simulink model "Echangeur_chaleur"  (R2020b)
settings: Solver=VariableStepAuto  StartTime=0.0  StopTime=10.0  RelTol=1e-3
values from neighbouring files (symbols this model uses):
  d_tube_big_ext = 0.106    [Conception_Preliminaire.m]    (also in Main.m)
  d_tube_big_int = 0.08    [Conception_Preliminaire.m]    (also in Main.m)
  d_tube_moy_ext = 0.01    [Conception_Preliminaire.m]    (also in Main.m)
  d_tube_moy_int = 0.007    [Conception_Preliminaire.m]    (also in Main.m)
  d_tube_small_ext = 0.006    [Conception_Preliminaire.m]    (also in Main.m)
  d_tube_small_int = 0.004    [Conception_Preliminaire.m]    (also in Main.m)
  h_int_MDI = 4.452    [Conception_Preliminaire.m]    (also in Main.m)
  k_acier = 36    [Conception_Preliminaire.m]    (also in Dimensionnement.m; Main.m)
  k_H2O = 0.147    [Conception_Preliminaire.m]    (also in Dimensionnement.m; Main.m)
  k_MDI = 0.08648    [Conception_Preliminaire.m]    (also in Dimensionnement.m; Main.m)
  L = 3    [Dimensionnement.m]    (also in Main.m = 2.72)
  Pr_H2O = 70    [Conception_Preliminaire.m]    (also in Main.m)
  Pr_lam_plaque_MDI = 10    [Conception_Preliminaire.m]    (also in Main.m)
  visc_H2O = 0.042    [Conception_Preliminaire.m]    (also in Dimensionnement.m; Main.m)
  visc_MDI = 0.19    [Conception_Preliminaire.m]    (also in Dimensionnement.m; Main.m)
settings Model: Creator=sam_f  LastModifiedBy=sam_f

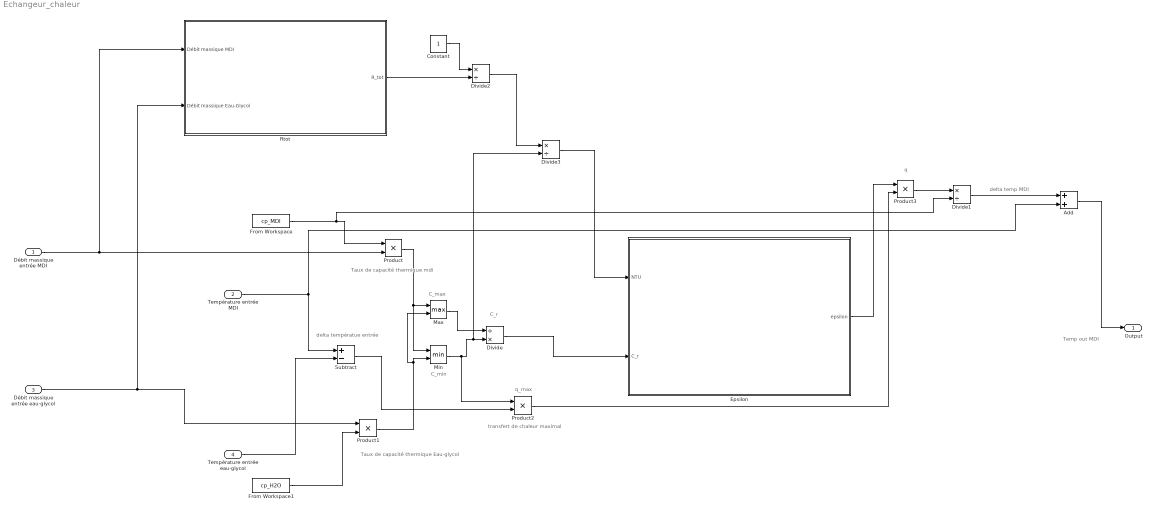
== system Echangeur_chaleur ==
  note: Temp out MDI
  note: delta temp MDI
  note: q
  note: transfert de chaleur maximal
  note: q_max
  note: delta températue entrée
  note: C_r
  note: C_max
  note: C_min
  note: Taux de capacité thermique mdi
  note: Taux de capacité thermique Eau-glycol
  Débit massique entrée MDI : Inport
  Température entrée MDI : Inport  Port=2
  Débit massique entrée eau-glycol : Inport  Port=3
  Température entrée eau-glycol : Inport  Port=4
  Add : Sum
  Constant : Constant
  Divide : Product  Inputs=/*
  Divide1 : Product  Inputs=*/
  Divide2 : Product  Inputs=*/
  Divide3 : Product  Inputs=*/
  Epsilon : Subsystem
  From Workspace : FromWorkspace  VariableName=cp_MDI
  From Workspace1 : FromWorkspace  VariableName=cp_H2O
  Max : MinMax  Function=max  Inputs=2
  Min : MinMax  Inputs=2
  Product{,1..3} (4 alike) : Product
  Rtot : Subsystem
  Subtract : Sum  Inputs=+-
  Output : Outport
  wires:
  Débit massique entrée MDI/1 -> Rtot/1(Débit massique MDI), Product/2
  From Workspace/1 -> Divide1/2, Product/1
  From Workspace1/1 -> Product1/2
  Product/1 -> Max/1, Min/1
  Product1/1 -> Max/2, Min/2
  Min/1 -> Product2/1, Divide3/2, Divide/2
  Max/1 -> Divide/1
  Divide/1 -> Epsilon/2(C_r)
  Température entrée MDI/1 -> Subtract/1, Add/2
  Subtract/1 -> Product2/2
  Débit massique entrée eau-glycol/1 -> Rtot/2(Débit massique Eau-Glycol), Product1/1
  Température entrée eau-glycol/1 -> Subtract/2
  Epsilon/1(epsilon) -> Product3/1
  Product2/1 -> Product3/2
  Product3/1 -> Divide1/1
  Divide1/1 -> Add/1
  Add/1 -> Output/1
  Constant/1 -> Divide2/1
  Divide2/1 -> Divide3/1
  Divide3/1 -> Epsilon/1(NTU)
  Rtot/1(R_tot) -> Divide2/2

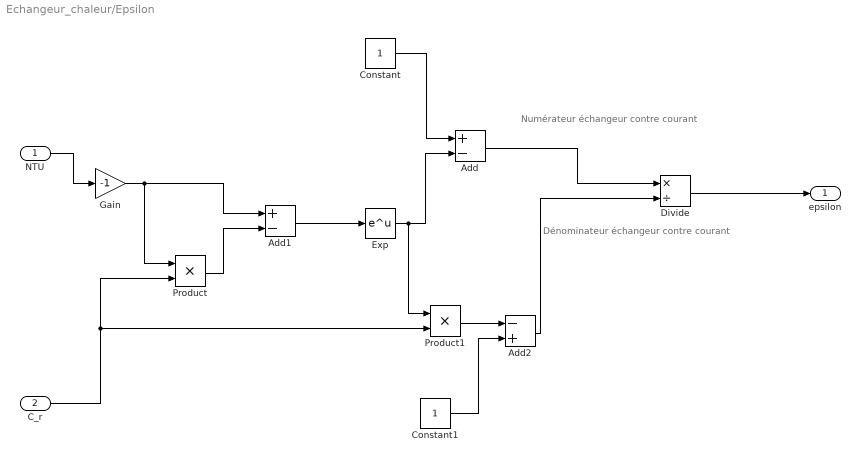
== system Echangeur_chaleur/Epsilon ==
  note: Numérateur échangeur contre courant
  note: Dénominateur échangeur contre courant
  NTU : Inport
  C_r : Inport  Port=2
  Add : Sum  Inputs=+-
  Add1 : Sum  Inputs=+-
  Add2 : Sum  Inputs=-+
  Constant : Constant
  Constant1 : Constant
  Divide : Product  Inputs=*/
  Exp : Math  SaturateOnIntegerOverflow=on
  Gain : Gain  Gain=-1
  Product : Product
  Product1 : Product
  epsilon : Outport
  wires:
  Divide/1 -> epsilon/1
  Add/1 -> Divide/1
  Constant/1 -> Add/1
  Exp/1 -> Product1/1, Add/2
  NTU/1 -> Gain/1
  Add1/1 -> Exp/1
  Gain/1 -> Product/1, Add1/1
  Product/1 -> Add1/2
  C_r/1 -> Product1/2, Product/2
  Add2/1 -> Divide/2
  Constant1/1 -> Add2/2
  Product1/1 -> Add2/1

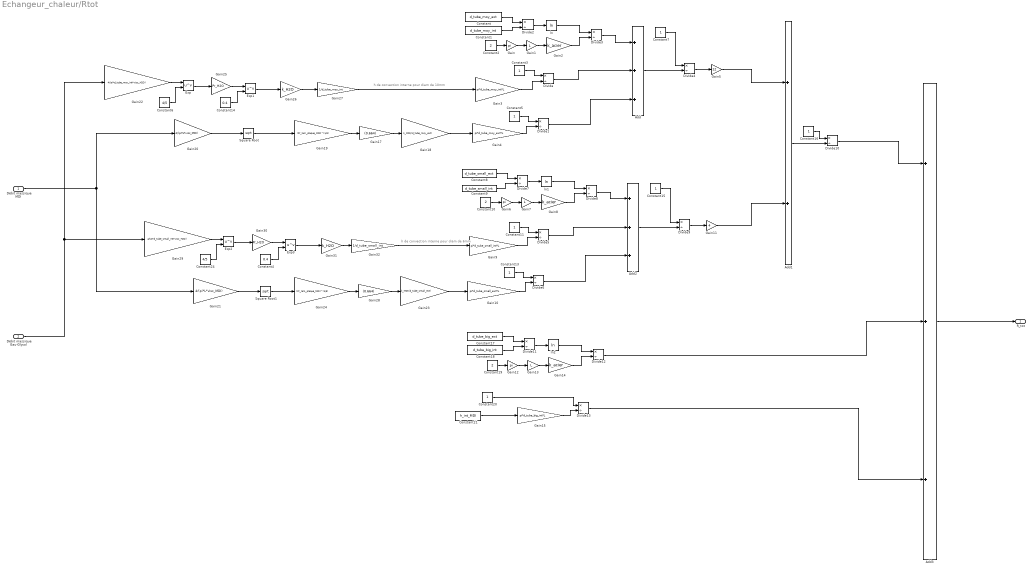
== system Echangeur_chaleur/Rtot ==
  note: h de convection interne pour diam de 10mm
  note: h de convection interne pour diam de 6mm
  Débit massique MDI : Inport
  Débit massique Eau-Glycol : Inport  Port=2
  Add : Sum  Inputs=+++
  Add1 : Sum
  Add2 : Sum  Inputs=+++
  Add3 : Sum  Inputs=+++
  Constant : Constant  Value=d_tube_moy_ext
  Constant1 : Constant  Value=d_tube_moy_int
  Constant10 : Constant  Value=2
  Constant{3,5,7,11,13,15..16,20} (8 alike) : Constant
  Constant14 : Constant  Value=0.4
  Constant17 : Constant  Value=d_tube_big_ext
  Constant18 : Constant  Value=d_tube_big_int
  Constant19 : Constant  Value=2
  Constant2 : Constant  Value=2
  Constant21 : Constant  Value=h_int_MDI
  Constant24 : Constant  Value=4/5
  Constant4 : Constant  Value=0.4
  Constant6 : Constant  Value=4/5
  Constant8 : Constant  Value=d_tube_small_ext
  Constant9 : Constant  Value=d_tube_small_int
  Divide{,1..13} (14 alike) : Product  Inputs=*/
  Exp{,1..3} (4 alike) : Math  Operator=pow  SaturateOnIntegerOverflow=on
  Gain : Gain  Gain=pi
  Gain1 : Gain  Gain=L
  Gain10 : Gain  Gain=pi*d_tube_small_ext*L
  Gain11 : Gain  Gain=4
  Gain12 : Gain  Gain=pi
  Gain13 : Gain  Gain=L
  Gain14 : Gain  Gain=k_acier
  Gain15 : Gain  Gain=pi*d_tube_big_int*L
  Gain17 : Gain  Gain=(0.664)
  Gain18 : Gain  Gain=k_MDI/(d_tube_moy_ext)
  Gain19 : Gain  Gain=(Pr_lam_plaque_MDI)^(1/3)
  Gain2 : Gain  Gain=k_acier
  Gain20 : Gain  Gain=4/(pi*L*visc_MDI)
  Gain21 : Gain  Gain=4/(pi*L*visc_MDI)
  Gain22 : Gain  Gain=4/(pi*d_tube_moy_int*visc_H2O)
  Gain23 : Gain  Gain=k_MDI/(d_tube_small_ext)
  Gain24 : Gain  Gain=(Pr_lam_plaque_MDI)^(1/3)
  Gain25 : Gain  Gain=Pr_H2O
  Gain26 : Gain  Gain=k_H2O
  Gain27 : Gain  Gain=1/d_tube_moy_int
  Gain28 : Gain  Gain=(0.664)
  Gain29 : Gain  Gain=4/(pi*d_tube_small_int*visc_H2O)
  Gain3 : Gain  Gain=pi*d_tube_moy_int*L
  Gain30 : Gain  Gain=Pr_H2O
  Gain31 : Gain  Gain=k_H2O
  Gain32 : Gain  Gain=1/d_tube_small_int
  Gain4 : Gain  Gain=pi*d_tube_moy_ext*L
  Gain5 : Gain  Gain=12
  Gain6 : Gain  Gain=pi
  Gain7 : Gain  Gain=L
  Gain8 : Gain  Gain=k_acier
  Gain9 : Gain  Gain=pi*d_tube_small_int*L
  Square Root : Sqrt  SaturateOnIntegerOverflow=on
  Square Root1 : Sqrt  SaturateOnIntegerOverflow=on
  ln : Math  Operator=log  SaturateOnIntegerOverflow=on
  ln1 : Math  Operator=log  SaturateOnIntegerOverflow=on
  ln2 : Math  Operator=log  SaturateOnIntegerOverflow=on
  R_tot : Outport
  wires:
  Gain1/1 -> Gain2/1
  Gain/1 -> Gain1/1
  Gain2/1 -> Divide3/2
  ln/1 -> Divide3/1
  Constant2/1 -> Gain/1
  Divide2/1 -> ln/1
  Constant1/1 -> Divide2/2
  Constant/1 -> Divide2/1
  Constant3/1 -> Divide/1
  Gain3/1 -> Divide/2
  Divide3/1 -> Add/1
  Divide/1 -> Add/2
  Divide1/1 -> Add/3
  Constant5/1 -> Divide1/1
  Gain4/1 -> Divide1/2
  Constant7/1 -> Divide4/1
  Add/1 -> Divide4/2
  Divide4/1 -> Gain5/1
  Gain5/1 -> Add1/1
  Divide9/1 -> Gain11/1
  Constant13/1 -> Divide6/1
  Constant15/1 -> Divide9/1
  Add2/1 -> Divide9/2
  Divide5/1 -> Add2/2
  Constant10/1 -> Gain6/1
  Gain6/1 -> Gain7/1
  Constant11/1 -> Divide5/1
  Divide7/1 -> ln1/1
  Constant9/1 -> Divide7/2
  Gain7/1 -> Gain8/1
  Gain10/1 -> Divide6/2
  Gain9/1 -> Divide5/2
  ln1/1 -> Divide8/1
  Divide8/1 -> Add2/1
  Gain8/1 -> Divide8/2
  Divide6/1 -> Add2/3
  Constant8/1 -> Divide7/1
  Gain11/1 -> Add1/2
  Constant16/1 -> Divide10/1
  Add1/1 -> Divide10/2
  Divide10/1 -> Add3/1
  Divide11/1 -> ln2/1
  Constant19/1 -> Gain12/1
  Gain12/1 -> Gain13/1
  Constant18/1 -> Divide11/2
  Gain13/1 -> Gain14/1
  ln2/1 -> Divide12/1
  Constant17/1 -> Divide11/1
  Gain14/1 -> Divide12/2
  Divide12/1 -> Add3/2
  Constant20/1 -> Divide13/1
  Constant21/1 -> Gain15/1
  Gain15/1 -> Divide13/2
  Divide13/1 -> Add3/3
  Add3/1 -> R_tot/1
  Gain17/1 -> Gain18/1
  Gain18/1 -> Gain4/1
  Gain19/1 -> Gain17/1
  Gain28/1 -> Gain23/1
  Gain24/1 -> Gain28/1
  Square Root/1 -> Gain19/1
  Gain20/1 -> Square Root/1
  Débit massique MDI/1 -> Gain21/1, Gain20/1
  Gain23/1 -> Gain10/1
  Square Root1/1 -> Gain24/1
  Gain21/1 -> Square Root1/1
  Gain22/1 -> Exp/1
  Constant6/1 -> Exp/2
  Débit massique Eau-Glycol/1 -> Gain29/1, Gain22/1
  Exp/1 -> Gain25/1
  Constant14/1 -> Exp1/2
  Gain25/1 -> Exp1/1
  Exp1/1 -> Gain26/1
  Gain26/1 -> Gain27/1
  Gain27/1 -> Gain3/1
  Gain30/1 -> Exp3/1
  Gain31/1 -> Gain32/1
  Exp3/1 -> Gain31/1
  Constant4/1 -> Exp3/2
  Constant24/1 -> Exp2/2
  Exp2/1 -> Gain30/1
  Gain29/1 -> Exp2/1
  Gain32/1 -> Gain9/1
